simulink model "Impedancias_diferentes_configuracoes_filtros"  (R2021a)
settings: Solver=ode23tb  StartTime=0.0  StopTime=10  RelTol=1e-6
InitFcn:
  | V_fund = 34.5e3
  | f_fund = 60
  | h_principal = 5*0.98
  | Q0 = 16
  | Q_filtro = 15e6
libraries: spsGroundLib x24, spsSeriesRLCBranchLib x24, spsImpedanceMeasurementLib x7, spsFourierLib x4, spsThreePhaseHarmonicFilterLib x3, spsACCurrentSourceLib x2, spsACVoltageSourceLib x2, spsCurrentMeasurementLib x2, spsVoltageMeasurementLib x2, spspowerguiLib x1
settings Model: Creator=angel  LastModifiedBy=angel
settings DebuggingCC: UnconnectedLineMsg=none

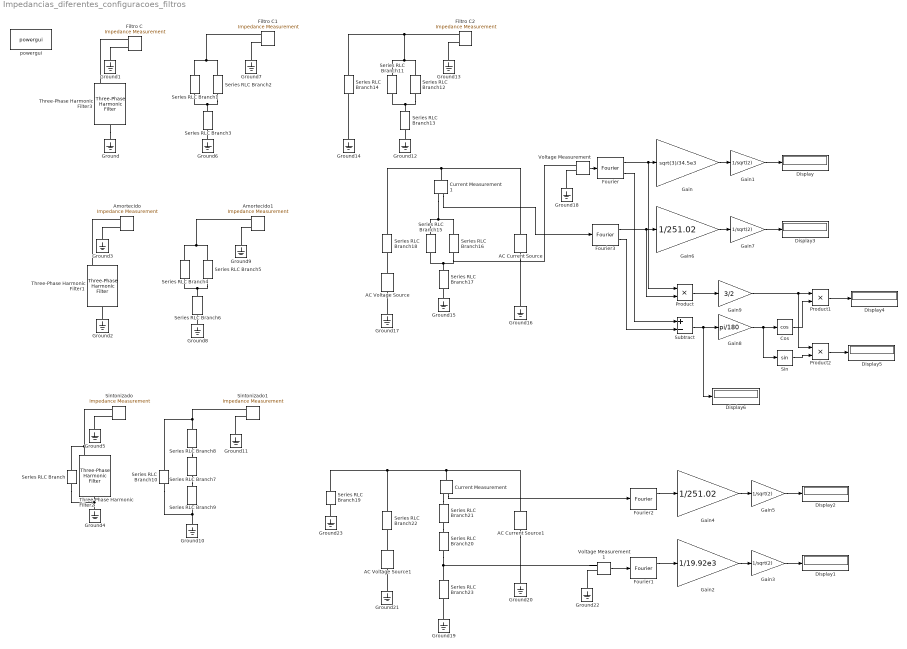
== system Impedancias_diferentes_configuracoes_filtros ==
  AC Current Source : spsACCurrentSourceLib/AC Current Source  Amplitude=sqrt(2)*500  Phase=0  Frequency=5*60  SampleTime=0  Measurements=None
      settings: SourceProductBaseCode=PS
  AC Current Source1 : spsACCurrentSourceLib/AC Current Source  Amplitude=sqrt(2)*500  Phase=0  Frequency=5*60  SampleTime=0  Measurements=None
      settings: SourceProductBaseCode=PS
  AC Voltage Source : spsACVoltageSourceLib/AC Voltage Source  Amplitude=sqrt(2)*34.5e3/sqrt(2)  Phase=0  Frequency=60  SampleTime=0  Measurements=None  BusType=swing  Pref=10e3  Qref=0  Qmin=-inf  Qmax=+inf
  AC Voltage Source1 : spsACVoltageSourceLib/AC Voltage Source  Amplitude=sqrt(2)*34.5e3/sqrt(3)  Phase=0  Frequency=60  SampleTime=0  Measurements=None  BusType=swing  Pref=10e3  Qref=0  Qmin=-inf  Qmax=+inf
  Amortecido : spsImpedanceMeasurementLib/Impedance Measurement  LConnTagsString=+|-  Factor=1
      settings: SourceProductBaseCode=PS
  Amortecido1 : spsImpedanceMeasurementLib/Impedance Measurement  LConnTagsString=+|-  Factor=1
      settings: SourceProductBaseCode=PS
  Cos : Trigonometry  Operator=cos
  Current Measurement : spsCurrentMeasurementLib/Current Measurement  PhasorSimulation=off  OutputType=Complex  PSBequivalent=0
  Current Measurement1 : spsCurrentMeasurementLib/Current Measurement  PhasorSimulation=off  OutputType=Complex  PSBequivalent=0
  Display{,1..6} (7 alike) : Display
  Filtro C : spsImpedanceMeasurementLib/Impedance Measurement  LConnTagsString=+|-  Factor=1
      settings: SourceProductBaseCode=PS
  Filtro C1 : spsImpedanceMeasurementLib/Impedance Measurement  LConnTagsString=+|-  Factor=1
      settings: SourceProductBaseCode=PS
  Filtro C2 : spsImpedanceMeasurementLib/Impedance Measurement  LConnTagsString=+|-  Factor=1
      settings: SourceProductBaseCode=PS
  Fourier : spsFourierLib/Fourier  Freq=60  n=5  InInit=[0, 0]  Ts=0
      settings: SourceProductBaseCode=PS
  Fourier1 : spsFourierLib/Fourier  Freq=60  n=5  InInit=[0, 0]  Ts=0
      settings: SourceProductBaseCode=PS
  Fourier2 : spsFourierLib/Fourier  Freq=60  n=1  InInit=[0, 0]  Ts=0
      settings: SourceProductBaseCode=PS
  Fourier3 : spsFourierLib/Fourier  Freq=60  n=5  InInit=[0, 0]  Ts=0
      settings: SourceProductBaseCode=PS
  Gain : Gain  Gain=sqrt(3)/34.5e3
  Gain{1,3,5,7} (4 alike) : Gain  Gain=1/sqrt(2)
  Gain2 : Gain  Gain=1/19.92e3
  Gain4 : Gain  Gain=1/251.02
  Gain6 : Gain  Gain=1/251.02
  Gain8 : Gain  Gain=pi/180
  Gain9 : Gain  Gain=3/2
  Ground{,1..23} (24 alike) : spsGroundLib/Ground  LConnTagsString=a
  Product : Product
  Product1 : Product
  Product2 : Product
  Series RLC Branch : spsSeriesRLCBranchLib/Series RLC Branch  LConnTagsString=__new0  RConnTagsString=__new0  BranchType=R  Resistance=1e6  Inductance=1e-3  SetiL0=off  InitialCurrent=0  Capacitance=1e-6  Setx0=off  InitialVoltage=0  Measurements=None
  Series RLC Branch1 : spsSeriesRLCBranchLib/Series RLC Branch  LConnTagsString=__new0  RConnTagsString=__new0  BranchType=LC  Resistance=1  Inductance=9.54e-3  SetiL0=off  InitialCurrent=0  Capacitance=737.16e-6  Setx0=off  InitialVoltage=0  Measurements=None
  Series RLC Branch10 : spsSeriesRLCBranchLib/Series RLC Branch  LConnTagsString=__new0  RConnTagsString=__new0  BranchType=R  Resistance=1e6  Inductance=1e-3  SetiL0=off  InitialCurrent=0  Capacitance=1e-6  Setx0=off  InitialVoltage=0  Measurements=None
  Series RLC Branch11 : spsSeriesRLCBranchLib/Series RLC Branch  LConnTagsString=__new0  RConnTagsString=__new0  BranchType=LC  Resistance=1  Inductance=9.54e-3  SetiL0=off  InitialCurrent=0  Capacitance=737.16e-6  Setx0=off  InitialVoltage=0  Measurements=None
  Series RLC Branch{2,5,12,16} (4 alike) : spsSeriesRLCBranchLib/Series RLC Branch  LConnTagsString=__new0  RConnTagsString=__new0  BranchType=R  Resistance=270.36  Inductance=9.54e-3  SetiL0=off  InitialCurrent=0  Capacitance=737.16e-6  Setx0=off  InitialVoltage=0  Measurements=None
  Series RLC Branch{3,6,9,13,17,23} (6 alike) : spsSeriesRLCBranchLib/Series RLC Branch  LConnTagsString=__new0  RConnTagsString=__new0  BranchType=C  Resistance=270.36  Inductance=9.54e-3  SetiL0=off  InitialCurrent=0  Capacitance=32.04e-6  Setx0=off  InitialVoltage=0  Measurements=None
  Series RLC Branch14 : spsSeriesRLCBranchLib/Series RLC Branch  LConnTagsString=__new0  RConnTagsString=__new0  BranchType=RL  Resistance=198.38e-3  Inductance=6.84e-3  SetiL0=off  InitialCurrent=0  Capacitance=737.16e-6  Setx0=off  InitialVoltage=0  Measurements=None
  Series RLC Branch15 : spsSeriesRLCBranchLib/Series RLC Branch  LConnTagsString=__new0  RConnTagsString=__new0  BranchType=LC  Resistance=1  Inductance=9.54e-3  SetiL0=off  InitialCurrent=0  Capacitance=737.16e-6  Setx0=off  InitialVoltage=0  Measurements=None
  Series RLC Branch18 : spsSeriesRLCBranchLib/Series RLC Branch  LConnTagsString=__new0  RConnTagsString=__new0  BranchType=RL  Resistance=198.38e-3  Inductance=6.84e-3  SetiL0=off  InitialCurrent=0  Capacitance=737.16e-6  Setx0=off  InitialVoltage=0  Measurements=None
  Series RLC Branch19 : spsSeriesRLCBranchLib/Series RLC Branch  LConnTagsString=__new0  RConnTagsString=__new0  BranchType=R  Resistance=1e6  Inductance=1e-3  SetiL0=off  InitialCurrent=0  Capacitance=1e-6  Setx0=off  InitialVoltage=0  Measurements=None
  Series RLC Branch20 : spsSeriesRLCBranchLib/Series RLC Branch  LConnTagsString=__new0  RConnTagsString=__new0  BranchType=L  Resistance=1  Inductance=9.15e-3  SetiL0=off  InitialCurrent=0  Capacitance=737.16e-6  Setx0=off  InitialVoltage=0  Measurements=None
  Series RLC Branch21 : spsSeriesRLCBranchLib/Series RLC Branch  LConnTagsString=__new0  RConnTagsString=__new0  BranchType=R  Resistance=1.06  Inductance=9.54e-3  SetiL0=off  InitialCurrent=0  Capacitance=737.16e-6  Setx0=off  InitialVoltage=0  Measurements=None
  Series RLC Branch22 : spsSeriesRLCBranchLib/Series RLC Branch  LConnTagsString=__new0  RConnTagsString=__new0  BranchType=RL  Resistance=198.38e-3  Inductance=6.84e-3  SetiL0=off  InitialCurrent=0  Capacitance=737.16e-6  Setx0=off  InitialVoltage=0  Measurements=None
  Series RLC Branch4 : spsSeriesRLCBranchLib/Series RLC Branch  LConnTagsString=__new0  RConnTagsString=__new0  BranchType=L  Resistance=1  Inductance=9.15e-3  SetiL0=off  InitialCurrent=0  Capacitance=737.16e-6  Setx0=off  InitialVoltage=0  Measurements=None
  Series RLC Branch7 : spsSeriesRLCBranchLib/Series RLC Branch  LConnTagsString=__new0  RConnTagsString=__new0  BranchType=L  Resistance=1  Inductance=9.15e-3  SetiL0=off  InitialCurrent=0  Capacitance=737.16e-6  Setx0=off  InitialVoltage=0  Measurements=None
  Series RLC Branch8 : spsSeriesRLCBranchLib/Series RLC Branch  LConnTagsString=__new0  RConnTagsString=__new0  BranchType=R  Resistance=1.06  Inductance=9.54e-3  SetiL0=off  InitialCurrent=0  Capacitance=737.16e-6  Setx0=off  InitialVoltage=0  Measurements=None
  Sin : Trigonometry
  Sintonizado : spsImpedanceMeasurementLib/Impedance Measurement  LConnTagsString=+|-  Factor=1
      settings: SourceProductBaseCode=PS
  Sintonizado1 : spsImpedanceMeasurementLib/Impedance Measurement  LConnTagsString=+|-  Factor=1
      settings: SourceProductBaseCode=PS
  Subtract : Sum  Inputs=+-
  Three-Phase Harmonic Filter1 : spsThreePhaseHarmonicFilterLib/Three-Phase Harmonic Filter  LConnTagsString=A|B|C  RConnTagsString=n  FilterType=High-pass  FilterConnection=Y (neutral)  ParNom=[V_fund f_fund]  Qc=Q_filtro  Fr=[h_principal*f_fund]  Frd=[11*60 13*60]  Q=Q0  Measurements=None
      settings: AttributesFormatString=\n  SourceProductBaseCode=PS
  Three-Phase Harmonic Filter2 : spsThreePhaseHarmonicFilterLib/Three-Phase Harmonic Filter  LConnTagsString=A|B|C  RConnTagsString=n  FilterType=Single-tuned  FilterConnection=Y (neutral)  ParNom=[V_fund f_fund]  Qc=Q_filtro  Fr=[h_principal*f_fund]  Frd=[11*60 13*60]  Q=Q0  Measurements=None
      settings: AttributesFormatString=\n  SourceProductBaseCode=PS
  Three-Phase Harmonic Filter3 : spsThreePhaseHarmonicFilterLib/Three-Phase Harmonic Filter  LConnTagsString=A|B|C  RConnTagsString=n  FilterType=C-type High-pass  FilterConnection=Y (neutral)  ParNom=[V_fund f_fund]  Qc=Q_filtro  Fr=[h_principal*f_fund]  Frd=[11*60 13*60]  Q=Q0  Measurements=None
      settings: AttributesFormatString=\n  SourceProductBaseCode=PS
  Voltage Measurement : spsVoltageMeasurementLib/Voltage Measurement  PhasorSimulation=off  OutputType=Complex  PSBequivalent=0
  Voltage Measurement1 : spsVoltageMeasurementLib/Voltage Measurement  PhasorSimulation=off  OutputType=Complex  PSBequivalent=0
  powergui : spspowerguiLib/powergui  Priority=1  SimulationMode=Continuous  SampleTime=50e-6  frequency=60  Iterations=50  frequencyindice=60  Pbase=100e6  ErrMax=1e-4  UnitsV=kV  UnitsW=MW  buscounter=0  FunctionMessages=off  echomessages=off  EnableUseOfTLC=off  CurrentSourceSwitches=off  DisableSnubberDevices=off  DisableRonSwitches=off  DisableVfSwitches=off  DisplayEquations=off  AutomaticDiscreteSolvers=off  SolverType=Tustin/Backward Euler (TBE)  Interpol=off  ExternalGateDelay=off  methode=off  Ts=100  x0status=blocks  SPID=on  SwTol=0  HookPort=off  NonlinearTolerance=1e-4  nMaxIteration=100  ContinueOnMaxIteration=off  RestoreLinks=warning  ResistiveCurrentMeasurement=off  Frange=[6:0.1:900]  Ylog=off  Xlog=off  ShowGrid=off  save=off  variable=ZData  structure=0  ZoomFFT=off  StartTime=0.0  cycles=1  DisplayStyle=1  fundamental=60  FreqAxis=off  MaxFrequency=1000  frequencyindicesteady=1  RmsSteady=1  display=off
  wires:
  Voltage Measurement/1 -> Fourier/1
  Fourier/1 -> Product/1, Gain/1
  Gain/1 -> Gain1/1
  Gain1/1 -> Display/1
  Gain3/1 -> Display1/1
  Gain2/1 -> Gain3/1
  Fourier1/1 -> Gain2/1
  Voltage Measurement1/1 -> Fourier1/1
  Fourier2/1 -> Gain4/1
  Gain4/1 -> Gain5/1
  Gain5/1 -> Display2/1
  Current Measurement/1 -> Fourier2/1
  Gain7/1 -> Display3/1
  Gain6/1 -> Gain7/1
  Fourier3/1 -> Product/2, Gain6/1
  Current Measurement1/1 -> Fourier3/1
  Subtract/1 -> Display6/1, Gain8/1
  Gain8/1 -> Sin/1, Cos/1
  Product/1 -> Gain9/1
  Cos/1 -> Product1/2
  Product1/1 -> Display4/1
  Sin/1 -> Product2/2
  Product2/1 -> Display5/1
  Gain9/1 -> Product2/1, Product1/1
  Fourier/2 -> Subtract/1
  Fourier3/2 -> Subtract/2
  connections:
  Three-Phase Harmonic Filter3/RConn1 -- Ground/LConn1
  Ground1/LConn1 -- Filtro C/LConn2
  Ground3/LConn1 -- Amortecido/LConn2
  Ground2/LConn1 -- Three-Phase Harmonic Filter1/RConn1
  Amortecido/LConn1 -- Three-Phase Harmonic Filter1/LConn1
  Sintonizado/LConn1 -- Series RLC Branch/LConn1 -- Three-Phase Harmonic Filter2/LConn1
  Ground4/LConn1 -- Series RLC Branch/RConn1 -- Three-Phase Harmonic Filter2/RConn1
  Ground5/LConn1 -- Sintonizado/LConn2
  Three-Phase Harmonic Filter3/LConn1 -- Filtro C/LConn1
  Series RLC Branch3/LConn1 -- Series RLC Branch2/RConn1 -- Series RLC Branch1/RConn1
  Series RLC Branch1/LConn1 -- Filtro C1/LConn1 -- Series RLC Branch2/LConn1
  Ground6/LConn1 -- Series RLC Branch3/RConn1
  Ground7/LConn1 -- Filtro C1/LConn2
  Series RLC Branch5/RConn1 -- Series RLC Branch6/LConn1 -- Series RLC Branch4/RConn1
  Amortecido1/LConn1 -- Series RLC Branch4/LConn1 -- Series RLC Branch5/LConn1
  Ground9/LConn1 -- Amortecido1/LConn2
  Ground8/LConn1 -- Series RLC Branch6/RConn1
  Ground11/LConn1 -- Sintonizado1/LConn2
  Ground10/LConn1 -- Series RLC Branch10/RConn1 -- Series RLC Branch9/RConn1
  Series RLC Branch7/RConn1 -- Series RLC Branch9/LConn1
  Series RLC Branch8/RConn1 -- Series RLC Branch7/LConn1
  Series RLC Branch8/LConn1 -- Series RLC Branch10/LConn1 -- Sintonizado1/LConn1
  Series RLC Branch12/RConn1 -- Series RLC Branch13/LConn1 -- Series RLC Branch11/RConn1
  Filtro C2/LConn1 -- Series RLC Branch14/LConn1 -- Series RLC Branch11/LConn1 -- Series RLC Branch12/LConn1
  Ground13/LConn1 -- Filtro C2/LConn2
  Ground12/LConn1 -- Series RLC Branch13/RConn1
  Ground14/LConn1 -- Series RLC Branch14/RConn1
  Series RLC Branch17/LConn1 -- Voltage Measurement/LConn1 -- Series RLC Branch16/RConn1 -- Series RLC Branch15/RConn1
  Series RLC Branch18/LConn1 -- Current Measurement1/LConn1 -- AC Current Source/RConn1
  AC Voltage Source/RConn1 -- Series RLC Branch18/RConn1
  Ground15/LConn1 -- Series RLC Branch17/RConn1
  AC Current Source/LConn1 -- Ground16/LConn1
  Ground18/LConn1 -- Voltage Measurement/LConn2
  Ground17/LConn1 -- AC Voltage Source/LConn1
  AC Current Source1/RConn1 -- Current Measurement/LConn1 -- Series RLC Branch19/LConn1 -- Series RLC Branch22/LConn1
  Ground21/LConn1 -- AC Voltage Source1/LConn1
  Ground22/LConn1 -- Voltage Measurement1/LConn2
  AC Voltage Source1/RConn1 -- Series RLC Branch22/RConn1
  AC Current Source1/LConn1 -- Ground20/LConn1
  Ground19/LConn1 -- Series RLC Branch23/RConn1
  Series RLC Branch20/RConn1 -- Voltage Measurement1/LConn1 -- Series RLC Branch23/LConn1
  Series RLC Branch21/RConn1 -- Series RLC Branch20/LConn1
  Ground23/LConn1 -- Series RLC Branch19/RConn1
  Current Measurement/RConn1 -- Series RLC Branch21/LConn1
  Series RLC Branch15/LConn1 -- Current Measurement1/RConn1 -- Series RLC Branch16/LConn1
